simulink model "ReactionPendulum_Simulation_Model"  (R2024b)
settings: Solver=ode23  StartTime=0.0  StopTime=50  MaxStep=1e-2  RelTol=1e-3
values from neighbouring files (symbols this model uses):
  fi_dc0 = 0    [currwork.mat]    (also in pendulum_friction_coefficient_identification.m)
  g = 9.81    [currwork.mat]    (also in pendulum_friction_coefficient_identification.m)
  J_pend = 0.026668518142893    (= 0.0266685181429)    [pendulum_friction_coefficient_identification.m]
  kr = 0.026    [currwork.mat]
  kt = 0.026    [currwork.mat]
  U = 0.012144    [currwork.mat]    (also in pendulum_friction_coefficient_identification.m)
  uc_dc = 0.0016    [currwork.mat]
  uc_pend = 0.00434561903982    [currwork.mat]    (also in pendulum_friction_coefficient_identification.m)
  uv_dc = 5.3017e-06    [currwork.mat]
  uv_pend = 0.000184765206116    [currwork.mat]    (also in pendulum_friction_coefficient_identification.m)
undefined symbols (not defined in the file or in its folder): J_dc, K, R_dc
settings Model: Creator=Student  LastModifiedBy=Paweł Wiktor
settings SolverCC: ZeroCrossAlgorithm=Adaptive  AlgebraicLoopSolver=TrustRegion
settings DataIOCC: ReturnWorkspaceOutputs=off
settings DebuggingCC: IgnoredZcDiagnostic=none  UnconnectedInputMsg=warning  UnconnectedOutputMsg=warning  UnconnectedLineMsg=warning  ArithmeticOperatorsInVariantConditions=warning
settings ModelReferenceCC: EnableRefExpFcnMdlSchedulingChecks=on
settings SFSimCC: CustomCodeUndefinedFunction=UseInterfaceOnly
settings RTWCC: GPUComputeCapability=3.5

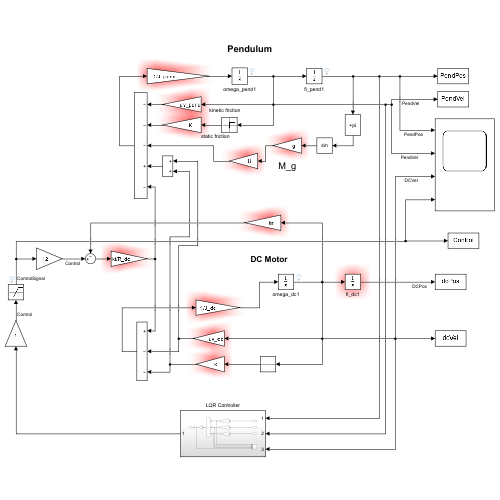
[thumbnail: Simulink's stored preview of the top-level diagram]
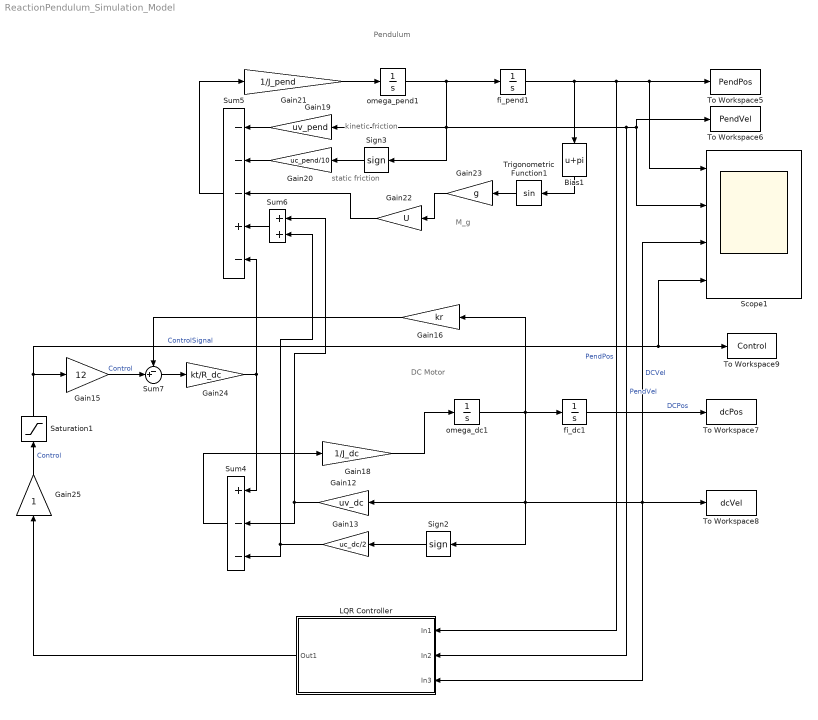
== system ReactionPendulum_Simulation_Model ==
  note: DC Motor
  note: kinetic friction
  note: Pendulum
  note: static friction
  note: M_g
  Bias1 : Bias  Bias=pi  SaturateOnIntegerOverflow=off
  Gain12 : Gain  Gain=uv_dc
  Gain13 : Gain  Gain=uc_dc/2
  Gain15 : Gain  Gain=12
  Gain16 : Gain  Gain=kr
  Gain18 : Gain  Gain=1/J_dc
  Gain19 : Gain  Gain=uv_pend
  Gain20 : Gain  Gain=uc_pend/10
  Gain21 : Gain  Gain=1/J_pend
  Gain22 : Gain  Gain=U
  Gain23 : Gain  Gain=g
  Gain24 : Gain  Gain=kt/R_dc
  Gain25 : Gain
  LQR Controller : Subsystem
  Saturation1 : Saturate  UpperLimit=1  LowerLimit=-1
  Scope1 : Scope  NumInputPorts=4
  Sign2 : Signum  ZeroCross=off
  Sign3 : Signum  ZeroCross=off
  Sum4 : Sum  Inputs=+--
  Sum5 : Sum  Inputs=---+-
  Sum6 : Sum
  Sum7 : Sum  Inputs=-+|
  To Workspace5 : ToWorkspace  VariableName=PendPos  SaveFormat=Structure With Time  SampleTime=-1
  To Workspace6 : ToWorkspace  VariableName=PendVel  SaveFormat=Structure With Time  SampleTime=-1
  To Workspace7 : ToWorkspace  VariableName=dcPos  SaveFormat=Structure With Time  SampleTime=-1
  To Workspace8 : ToWorkspace  VariableName=dcVel  SaveFormat=Structure With Time  SampleTime=-1
  To Workspace9 : ToWorkspace  VariableName=Control  SaveFormat=Structure With Time  SampleTime=-1
  Trigonometric Function1 : Trigonometry
  fi_dc1 : Integrator  InitialCondition=fi_dc0
  fi_pend1 : Integrator  InitialCondition=deg2rad(30)
  omega_dc1 : Integrator  InitialCondition=0%deg2rad(25000)
  omega_pend1 : Integrator  InitialCondition=0%deg2rad(30)
  wires:
  fi_pend1/1 -> LQR Controller/1(In1), Scope1/1, To Workspace5/1, Bias1/1  "PendPos"
  Sum4/1 -> Gain18/1
  Bias1/1 -> Trigonometric Function1/1
  Gain20/1 -> Sum5/2
  Gain25/1 -> Saturation1/1  "Control"
  Trigonometric Function1/1 -> Gain23/1
  Gain18/1 -> omega_dc1/1
  Gain15/1 -> Sum7/2  "Control"
  omega_pend1/1 -> Sign3/1, LQR Controller/2(In2), To Workspace6/1, Scope1/2, Gain19/1, fi_pend1/1  "PendVel"
  Sum7/1 -> Gain24/1
  Gain21/1 -> omega_pend1/1
  LQR Controller/1(Out1) -> Gain25/1
  Saturation1/1 -> Scope1/4, To Workspace9/1, Gain15/1  "ControlSignal"
  Gain16/1 -> Sum7/1
  Sum6/1 -> Sum5/4
  Gain12/1 -> Sum4/2, Sum6/1
  Sign2/1 -> Gain13/1
  Gain23/1 -> Gain22/1
  omega_dc1/1 -> Gain16/1, fi_dc1/1, Scope1/3, To Workspace8/1, LQR Controller/3(In3), Sign2/1, Gain12/1  "DCVel"
  Sum5/1 -> Gain21/1
  fi_dc1/1 -> To Workspace7/1  "DCPos"
  Gain24/1 -> Sum5/5, Sum4/1
  Gain22/1 -> Sum5/3
  Gain13/1 -> Sum4/3, Sum6/2
  Sign3/1 -> Gain20/1
  Gain19/1 -> Sum5/1

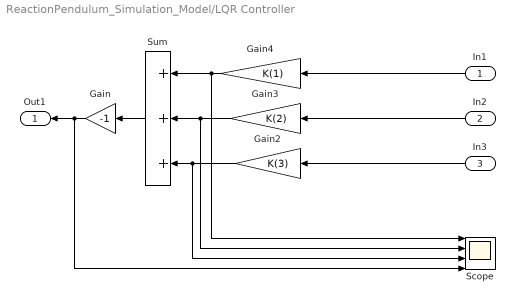
== system ReactionPendulum_Simulation_Model/LQR Controller ==
  In1 : Inport
  In2 : Inport  Port=2
  In3 : Inport  Port=3
  Gain : Gain  Gain=-1
  Gain2 : Gain  Gain=K(3)
  Gain3 : Gain  Gain=K(2)
  Gain4 : Gain  Gain=K(1)
  Scope : Scope  NumInputPorts=4
  Sum : Sum  Inputs=+++
  Out1 : Outport  VectorParamsAs1DForOutWhenUnconnected=off
  wires:
  In1/1 -> Gain4/1
  In2/1 -> Gain3/1
  In3/1 -> Gain2/1
  Gain2/1 -> Scope/3, Sum/3
  Gain3/1 -> Scope/2, Sum/2
  Gain4/1 -> Scope/1, Sum/1
  Sum/1 -> Gain/1
  Gain/1 -> Scope/4, Out1/1
